simulink model "Project4"  (R2016a)
settings: Solver=ode5  StartTime=0.0  StopTime=10.0  FixedStep=0.001  RelTol=1e-3
values from neighbouring files (symbols this model uses):
  a1_c = 1.5    [Project4_Code.m]
  a2_c = 2    [Project4_Code.m]
  b_c = 5.5    [Project4_Code.m]
  beta = sqrt(b_upp/b_low)    [Project4_Code.m]
  bhat_inv = 1/bhat    [Project4_Code.m]
  const_para_sw = 0    [Project4_Code.m]
  ita = 0.1    [Project4_Code.m]
  lambda = 20    [Project4_Code.m]
  phi = 0.1    [Project4_Code.m]
  signum_sw = 1    [Project4_Code.m]
  x0 = 0    [Project4_Code.m]
  xdot0 = pi/2    (= 1.57079632679)    [Project4_Code.m]
settings Model: Creator=Dell  LastModifiedBy=Dell

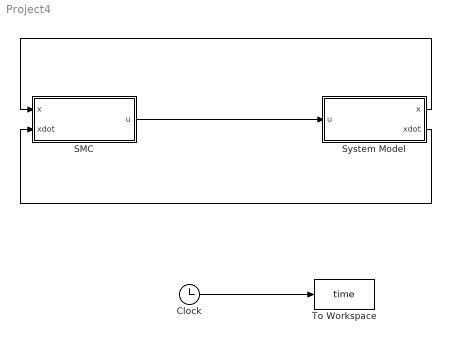
== system Project4 ==
  Clock : Clock
  SMC : Subsystem
  System Model : Subsystem
  To Workspace : ToWorkspace  VariableName=time  SampleTime=-1
  wires:
  System Model/1(x) -> SMC/1(x)
  System Model/2(xdot) -> SMC/2(xdot)
  Clock/1 -> To Workspace/1
  SMC/1(u) -> System Model/1(u)

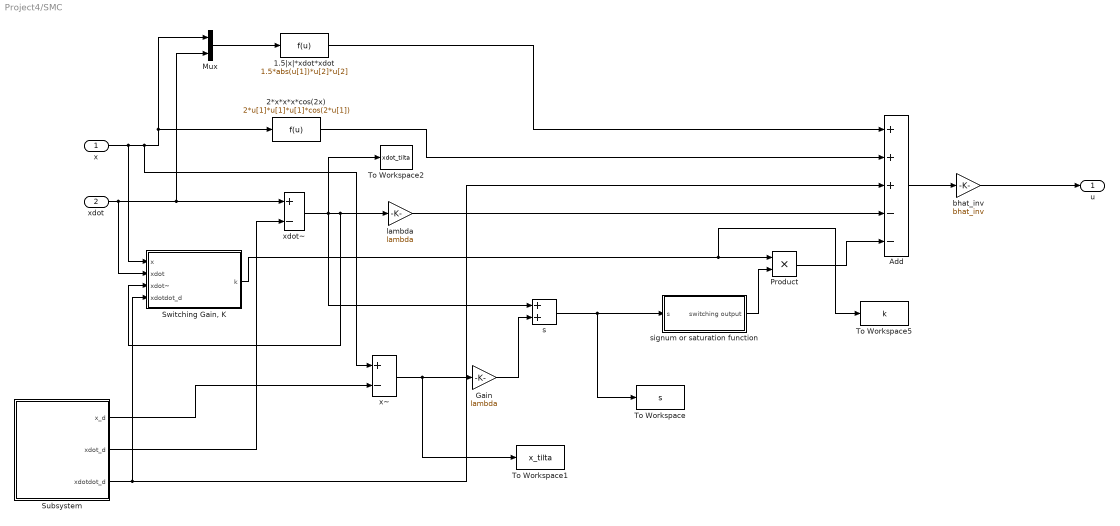
== system Project4/SMC ==
  x : Inport
  xdot : Inport  Port=2
  1.5|x|*xdot*xdot : Fcn  Expr=1.5*abs(u[1])*u[2]*u[2]
  2*x*x*x*cos(2x) : Fcn  Expr=2*u[1]*u[1]*u[1]*cos(2*u[1])
  Add : Sum  Inputs=+++--
  Gain : Gain  Gain=lambda
  Mux : Mux  Inputs=2
  Product : Product
  Subsystem : Subsystem
  "Switching Gain, K" : Subsystem
  To Workspace : ToWorkspace  VariableName=s  SampleTime=-1
  To Workspace1 : ToWorkspace  VariableName=x_tilta  SampleTime=-1
  To Workspace2 : ToWorkspace  VariableName=xdot_tilta  SampleTime=-1
  To Workspace5 : ToWorkspace  VariableName=k  SampleTime=-1
  bhat_inv : Gain  Gain=bhat_inv
  lambda : Gain  Gain=lambda
  s : Sum
  signum or saturation function : Subsystem
  xdot~ : Sum  Inputs=+-
  x~ : Sum  Inputs=+-
  u : Outport
  wires:
  x/1 -> "Switching Gain, K"/1(x), x~/1, 2*x*x*x*cos(2x)/1, Mux/1
  xdot/1 -> "Switching Gain, K"/2(xdot), xdot~/1, Mux/2
  Mux/1 -> 1.5|x|*xdot*xdot/1
  1.5|x|*xdot*xdot/1 -> Add/1
  2*x*x*x*cos(2x)/1 -> Add/2
  Subsystem/3(xdotdot_d) -> "Switching Gain, K"/4(xdotdot_d), Add/3
  Subsystem/2(xdot_d) -> xdot~/2
  xdot~/1 -> s/1, To Workspace2/1, "Switching Gain, K"/3(xdot~), lambda/1
  lambda/1 -> Add/4
  Subsystem/1(x_d) -> x~/2
  x~/1 -> To Workspace1/1, Gain/1
  Gain/1 -> s/2
  s/1 -> To Workspace/1, signum or saturation function/1(s)
  signum or saturation function/1(switching output) -> Product/2
  "Switching Gain, K"/1(k) -> Product/1, To Workspace5/1
  Product/1 -> Add/5
  Add/1 -> bhat_inv/1
  bhat_inv/1 -> u/1

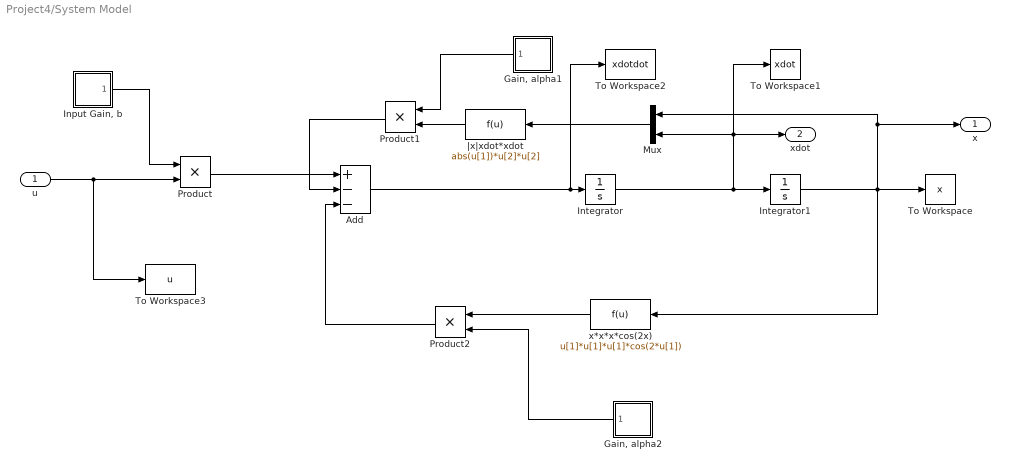
== system Project4/System Model ==
  u : Inport
  Add : Sum  Inputs=+--
  "Gain, alpha1" : Subsystem
  "Gain, alpha2" : Subsystem
  "Input Gain, b" : Subsystem
  Integrator : Integrator  InitialCondition=xdot0
  Integrator1 : Integrator  InitialCondition=x0
  Mux : Mux  Inputs=2
  Product : Product
  Product1 : Product
  Product2 : Product
  To Workspace : ToWorkspace  VariableName=x  SampleTime=-1
  To Workspace1 : ToWorkspace  VariableName=xdot  SampleTime=-1
  To Workspace2 : ToWorkspace  VariableName=xdotdot  SampleTime=-1
  To Workspace3 : ToWorkspace  VariableName=u  SampleTime=-1
  x*x*x*cos(2x) : Fcn  Expr=u[1]*u[1]*u[1]*cos(2*u[1])
  |x|xdot*xdot : Fcn  Expr=abs(u[1])*u[2]*u[2]
  x : Outport
  xdot : Outport  Port=2
  wires:
  u/1 -> To Workspace3/1, Product/2
  "Input Gain, b"/1(Out1) -> Product/1
  Product/1 -> Add/1
  Integrator/1 -> To Workspace1/1, xdot/1, Mux/2, Integrator1/1
  Add/1 -> To Workspace2/1, Integrator/1
  Integrator1/1 -> x*x*x*cos(2x)/1, Mux/1, x/1, To Workspace/1
  Mux/1 -> |x|xdot*xdot/1
  |x|xdot*xdot/1 -> Product1/2
  "Gain, alpha1"/1(Out1) -> Product1/1
  Product1/1 -> Add/2
  x*x*x*cos(2x)/1 -> Product2/1
  "Gain, alpha2"/1(Out1) -> Product2/2
  Product2/1 -> Add/3

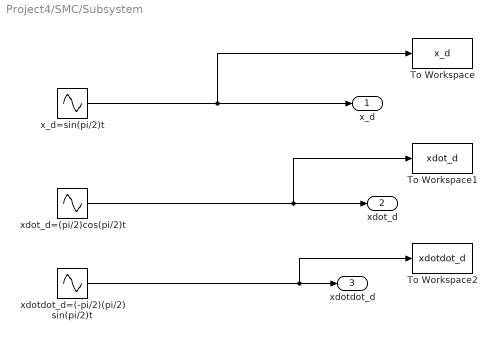
== system Project4/SMC/Subsystem ==
  To Workspace : ToWorkspace  VariableName=x_d  SampleTime=-1
  To Workspace1 : ToWorkspace  VariableName=xdot_d  SampleTime=-1
  To Workspace2 : ToWorkspace  VariableName=xdotdot_d  SampleTime=-1
  x_d=sin(pi/2)t : Sin  Frequency=pi/2  SampleTime=0
  xdot_d=(pi/2)cos(pi/2)t : Sin  Amplitude=pi/2  Frequency=pi/2  Phase=pi/2  SampleTime=0
  xdotdot_d=(-pi/2)(pi/2)sin(pi/2)t : Sin  Amplitude=-(pi/2)*(pi/2)  Frequency=pi/2  SampleTime=0
  x_d : Outport
  xdot_d : Outport  Port=2
  xdotdot_d : Outport  Port=3
  wires:
  x_d=sin(pi/2)t/1 -> To Workspace/1, x_d/1
  xdot_d=(pi/2)cos(pi/2)t/1 -> To Workspace1/1, xdot_d/1
  xdotdot_d=(-pi/2)(pi/2)sin(pi/2)t/1 -> To Workspace2/1, xdotdot_d/1

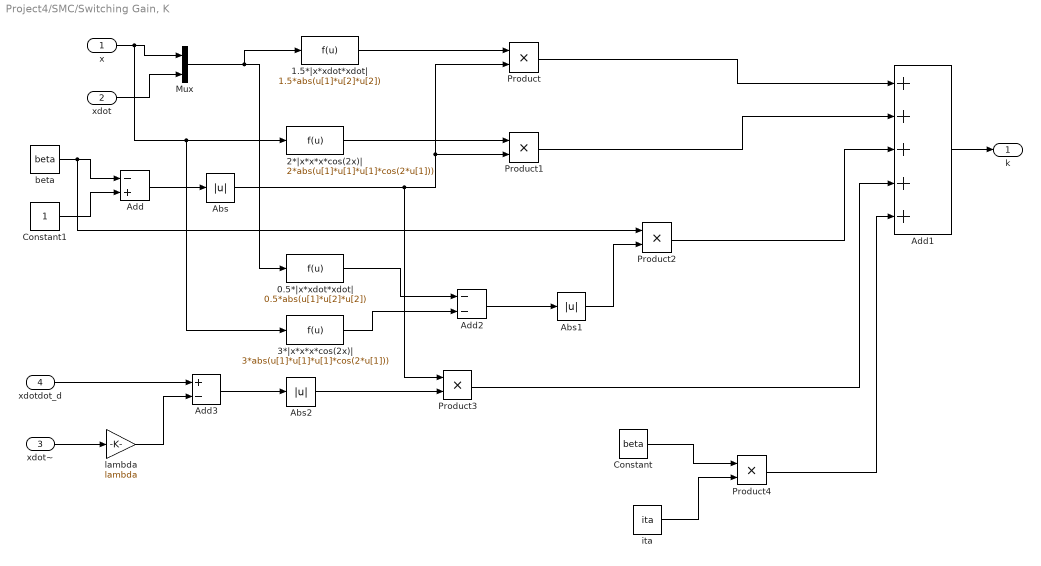
== system Project4/SMC/Switching Gain, K ==
  x : Inport
  xdot : Inport  Port=2
  xdot~ : Inport  Port=3
  xdotdot_d : Inport  Port=4
  0.5*|x*xdot*xdot| : Fcn  Expr=0.5*abs(u[1]*u[2]*u[2])
  1.5*|x*xdot*xdot| : Fcn  Expr=1.5*abs(u[1]*u[2]*u[2])
  2*|x*x*x*cos(2x)| : Fcn  Expr=2*abs(u[1]*u[1]*u[1]*cos(2*u[1]))
  3*|x*x*x*cos(2x)| : Fcn  Expr=3*abs(u[1]*u[1]*u[1]*cos(2*u[1]))
  Abs : Abs
  Abs1 : Abs
  Abs2 : Abs
  Add : Sum  Inputs=-+
  Add1 : Sum  Inputs=+++++
  Add2 : Sum  Inputs=--
  Add3 : Sum  Inputs=+-
  Constant : Constant  Value=beta
  Constant1 : Constant
  Mux : Mux  Inputs=2
  Product{,1..4} (5 alike) : Product
  beta : Constant  Value=beta
  ita : Constant  Value=ita
  lambda : Gain  Gain=lambda
  k : Outport
  wires:
  x/1 -> 3*|x*x*x*cos(2x)|/1, 2*|x*x*x*cos(2x)|/1, Mux/1
  xdot/1 -> Mux/2
  beta/1 -> Product2/1, Add/1
  Constant1/1 -> Add/2
  Add/1 -> Abs/1
  Mux/1 -> 0.5*|x*xdot*xdot|/1, 1.5*|x*xdot*xdot|/1
  1.5*|x*xdot*xdot|/1 -> Product/1
  Abs/1 -> Product3/1, Product1/2, Product/2
  Product/1 -> Add1/1
  2*|x*x*x*cos(2x)|/1 -> Product1/1
  Product1/1 -> Add1/2
  0.5*|x*xdot*xdot|/1 -> Add2/1
  3*|x*x*x*cos(2x)|/1 -> Add2/2
  Add2/1 -> Abs1/1
  Abs1/1 -> Product2/2
  Product2/1 -> Add1/3
  xdot~/1 -> lambda/1
  xdotdot_d/1 -> Add3/1
  lambda/1 -> Add3/2
  Add3/1 -> Abs2/1
  Abs2/1 -> Product3/2
  Product3/1 -> Add1/4
  Constant/1 -> Product4/1
  ita/1 -> Product4/2
  Product4/1 -> Add1/5
  Add1/1 -> k/1

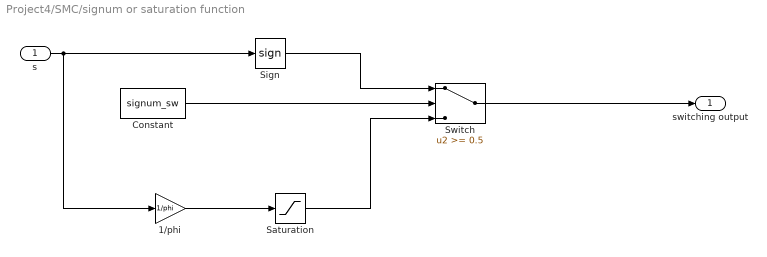
== system Project4/SMC/signum or saturation function ==
  s : Inport
  1/phi : Gain  Gain=1/phi
  Constant : Constant  Value=signum_sw
  Saturation : Saturate  UpperLimit=1  LowerLimit=-1
  Sign : Signum
  Switch : Switch  Threshold=0.5
  switching output : Outport
  wires:
  s/1 -> 1/phi/1, Sign/1
  Sign/1 -> Switch/1
  Constant/1 -> Switch/2
  1/phi/1 -> Saturation/1
  Saturation/1 -> Switch/3
  Switch/1 -> switching output/1

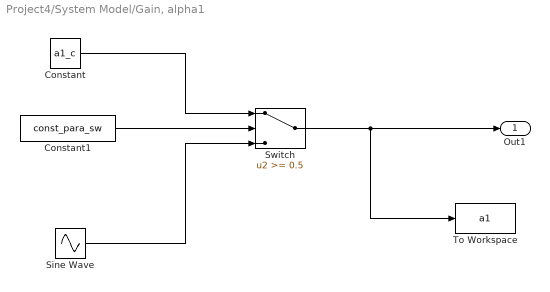
== system Project4/System Model/Gain, alpha1 ==
  Constant : Constant  Value=a1_c
  Constant1 : Constant  Value=const_para_sw
  Sine Wave : Sin  Amplitude=0.5  Bias=1.5  SampleTime=0
  Switch : Switch  Threshold=0.5
  To Workspace : ToWorkspace  VariableName=a1  SampleTime=-1
  Out1 : Outport
  wires:
  Constant1/1 -> Switch/2
  Constant/1 -> Switch/1
  Sine Wave/1 -> Switch/3
  Switch/1 -> To Workspace/1, Out1/1

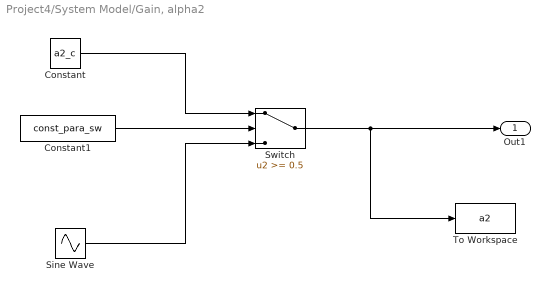
== system Project4/System Model/Gain, alpha2 ==
  Constant : Constant  Value=a2_c
  Constant1 : Constant  Value=const_para_sw
  Sine Wave : Sin  Amplitude=3  Bias=2  SampleTime=0
  Switch : Switch  Threshold=0.5
  To Workspace : ToWorkspace  VariableName=a2  SampleTime=-1
  Out1 : Outport
  wires:
  Constant1/1 -> Switch/2
  Constant/1 -> Switch/1
  Sine Wave/1 -> Switch/3
  Switch/1 -> To Workspace/1, Out1/1

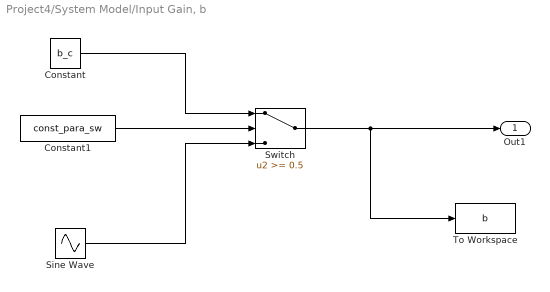
== system Project4/System Model/Input Gain, b ==
  Constant : Constant  Value=b_c
  Constant1 : Constant  Value=const_para_sw
  Sine Wave : Sin  Amplitude=1.5  Bias=5.5  SampleTime=0
  Switch : Switch  Threshold=0.5
  To Workspace : ToWorkspace  VariableName=b  SampleTime=-1
  Out1 : Outport
  wires:
  Constant1/1 -> Switch/2
  Constant/1 -> Switch/1
  Sine Wave/1 -> Switch/3
  Switch/1 -> To Workspace/1, Out1/1
